simulink model "buffer_m"  (Simulink 7.9)
settings: Solver=ode45  SolverMode=SingleTasking  StartTime=0.0  StopTime=999999  MaxStep=10  RelTol=1e-3  AbsTol=1e-3
values from neighbouring files (symbols this model uses):
  U = st_Varia('LongNames')    [buffWQ_i.m]    (also in buffal_i.m; buffer_i.m)
  x0 = zeros(U.Number,1)    [buffWQ_i.m]    (also in buffWQ_s.m = x0; buffal_i.m; buffal_s.m = x0; buffer_s.m = x0)
undefined symbols (not defined in the file or in its folder): B
settings Model: Creator=M.Sparnaaij  LastModifiedBy=M.Sparnaaij
settings DataIOCC: LimitDataPoints=off  SaveOutput=off  SaveTime=off  SignalLoggingName=sigsOut
settings OptimizationCC: BooleanDataType=off
settings DebuggingCC: SaveWithParameterizedLinksMsg=none  SignalResolutionControl=TryResolveAllWithWarning  SolverPrmCheckMsg=none  MultiTaskDSMMsg=warning  MultiTaskCondExecSysMsg=none  StrictBusMsg=None
settings HardwareCC: TargetUnknown=on
settings RTWCC: IncludeERTFirstTime=on
settings GRTTargetCC: CombineOutputUpdateFcns=off  GRTInterface=on

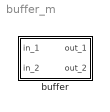
== system buffer_m ==
  buffer : Subsystem  Description=buffer
      mask init:
      | filenaam='.\StimelaData\buffer_p.mat';
      | 
      | [Pn,Fn,Fext]=Fileprop(filenaam);
      | 
      | errstr = st_UniqName(filenaam,'filenaam=''','SubSystem','OpenFcn');
      | if errstr, error([errstr 'The filename "' filenaam '" is already in use. Choose a different filename.']), end
      | 
      | P = buffer_p(filenaam);
      | [B,x0,U]=buffer_i(filenaam);
      settings: OpenFcn=|
      | filenaam='.\StimelaData\buffer_p.mat';
      | st_ParameterInput('init',gcb,filenaam,'buffer');
      mask Display:
      | plot(0,0,100,100,[0 20],[80 80],[0 20],[85 85],[0 20],[20 20],[80 100],[80 80],[80 100],[85 85],[80 100],[ 20 20],[20 80 80 20 20],[10 10 90  90 10]);
      | disp('')
      | text(50,50,'buffer', 'horizontalAlignment', 'center', 'verticalAlignment', 'middle');
      | text(50,0,Fn, 'horizontalAlignment', 'center', 'verticalAlignment', 'base');

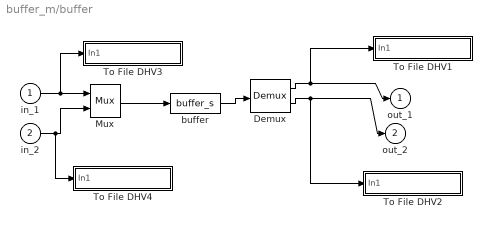
== system buffer_m/buffer ==
  in_1 : Inport
  in_2 : Inport  Port=2
  Demux : Demux  Outputs=[U.Number B.Measurements]
  Mux : Mux  Inputs=[U.Number B.Setpoints]
  To File DHV1 : Subsystem  mask(To File DHV){naam=[filenaam(1:length(filenaam)-4) '_out.sti']}
      mask prompts: naam "Naam van bestand"
      mask init:
      | set_param([gcb '/To File'],'Filename',naam);
      mask Display: disp(naam)
  To File DHV2 : Subsystem  mask(To File DHV){naam=[filenaam(1:length(filenaam)-4) '_EM.sti']}
      mask prompts: naam "Naam van bestand"
      mask init:
      | set_param([gcb '/To File'],'Filename',naam);
      mask Display: disp(naam)
  To File DHV3 : Subsystem  mask(To File DHV){naam=[filenaam(1:length(filenaam)-4) '_in.sti']}
      mask prompts: naam "Naam van bestand"
      mask init:
      | set_param([gcb '/To File'],'Filename',naam);
      mask Display: disp(naam)
  To File DHV4 : Subsystem  mask(To File DHV){naam=[filenaam(1:length(filenaam)-4) '_ES.sti']}
      mask prompts: naam "Naam van bestand"
      mask init:
      | set_param([gcb '/To File'],'Filename',naam);
      mask Display: disp(naam)
  buffer : S-Function  FunctionName=buffer_s  Parameters=B,x0,U,P  EnableBusSupport=off
  out_1 : Outport  InitialOutput=0
  out_2 : Outport  Port=2  InitialOutput=0
  wires:
  in_2/1 -> To File DHV4/1(In1), Mux/2
  Mux/1 -> buffer/1
  in_1/1 -> To File DHV3/1(In1), Mux/1
  buffer/1 -> Demux/1
  Demux/1 -> To File DHV1/1(In1), out_1/1
  Demux/2 -> To File DHV2/1(In1), out_2/1

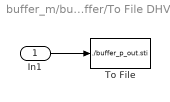
== system buffer_m/buffer/To File DHV1 ==
  In1 : Inport
  To File : ToFile  Filename=./buffer_p_out.sti  MatrixName=bufferout
  wires:
  In1/1 -> To File/1

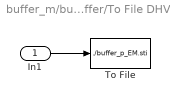
== system buffer_m/buffer/To File DHV2 ==
  In1 : Inport
  To File : ToFile  Filename=./buffer_p_EM.sti  MatrixName=bufferEM
  wires:
  In1/1 -> To File/1

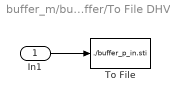
== system buffer_m/buffer/To File DHV3 ==
  In1 : Inport
  To File : ToFile  Filename=./buffer_p_in.sti  MatrixName=bufferin
  wires:
  In1/1 -> To File/1

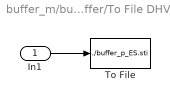
== system buffer_m/buffer/To File DHV4 ==
  In1 : Inport
  To File : ToFile  Filename=./buffer_p_ES.sti  MatrixName=bufferES
  wires:
  In1/1 -> To File/1
